simulink model "real_LAB4"  (R2025b)
settings: Solver=VariableStepAuto  StartTime=0.0  StopTime=10.0  RelTol=1e-3
undefined symbols (not defined in the file or in its folder): C, DiscIntNeverNeededParam, drv, gbox, K, K_e, Nu, Nx, sens, Tc, Ts, wheel
settings Model: Creator=ester  LastModifiedBy=ester

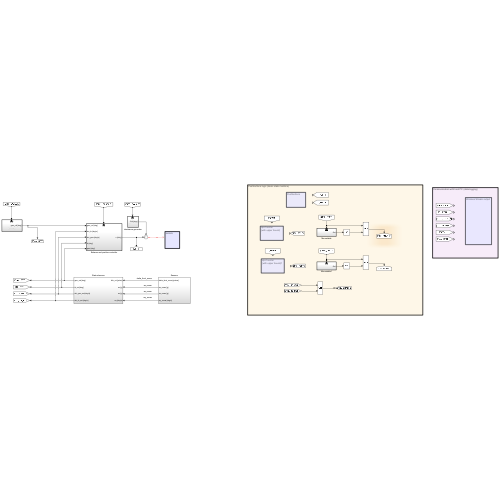
[thumbnail: Simulink's stored preview of the top-level diagram]
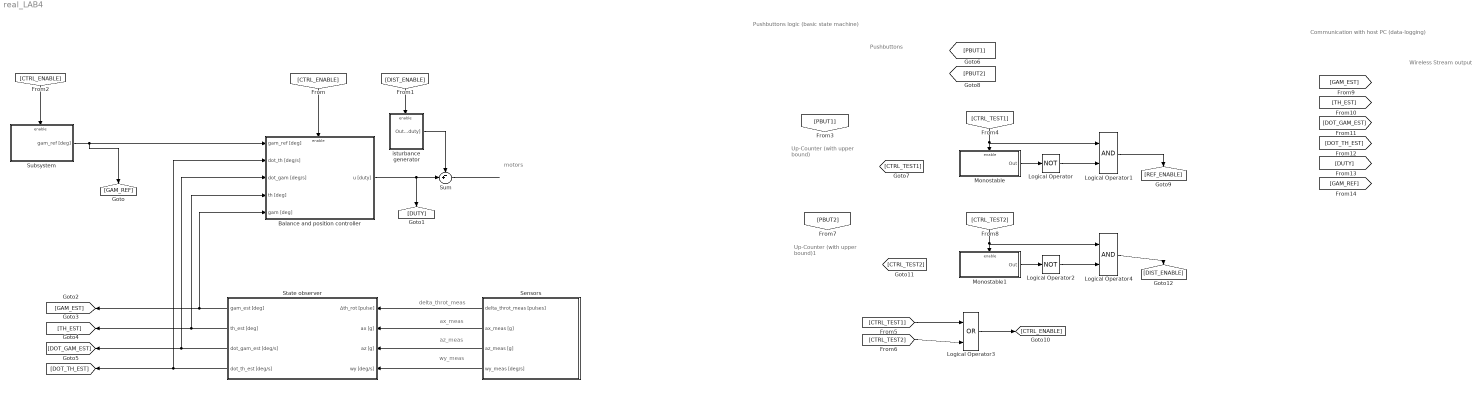
== system real_LAB4 ==
  note: Communication with host PC (data-logging)
  note: Wireless Stream output
  note: Pushbuttons logic (basic state machine)
  note: Up-Counter
      | (with upper bound)
  note: Pushbuttons
  note: motors
  note: ax_meas
  note: delta_throt_meas
  note: az_meas
  note: wy_meas
  note: Up-Counter
      | (with upper bound)1
  Balance and position controller : Subsystem
  Logical Operator : Logic  Operator=NOT  AllPortsSameDT=off  OutDataTypeStr=boolean
  Logical Operator1 : Logic  AllPortsSameDT=off  OutDataTypeStr=boolean
  Logical Operator2 : Logic  Operator=NOT  AllPortsSameDT=off  OutDataTypeStr=boolean
  Logical Operator3 : Logic  Operator=OR  AllPortsSameDT=off  OutDataTypeStr=boolean
  Logical Operator4 : Logic  AllPortsSameDT=off  OutDataTypeStr=boolean
  Monostable : Subsystem
  Monostable1 : Subsystem
  Sensors : Subsystem
  State observer : Subsystem
  Subsystem : Subsystem
  Sum : Sum  Inputs=-+|
  isturbance generator : Subsystem
  wires:
  Subsystem/1(gam_ref [deg]) -> [GAM_REF], Balance and position controller/1(gam_ref [deg])
  Balance and position controller/1(u [duty]) -> [DUTY], Sum/2
  isturbance generator/1(Out [duty]) -> Sum/1
  [DIST_ENABLE] -> isturbance generator/Enable
  [CTRL_ENABLE] -> Subsystem/Enable
  [CTRL_ENABLE] -> Balance and position controller/Enable
  Sum/1 -> ?
  Sensors/3(az_meas [g]) -> State observer/3(az [g])
  Sensors/4(wy_meas [deg/s]) -> State observer/4(wy [deg/s])
  Sensors/2(ax_meas [g]) -> State observer/2(ax [g])
  Sensors/1(delta_throt_meas [pulses]) -> State observer/1(Δth_rot [pulse])
  State observer/2(th_est [deg]) -> [TH_EST], Balance and position controller/4(th [deg])
  State observer/3(dot_gam_est [deg/s]) -> Balance and position controller/3(dot_gam [deg/s]), [DOT_GAM_EST]
  State observer/4(dot_th_est [deg/s]) -> [DOT_TH_EST], Balance and position controller/2(dot_th [deg/s])
  [CTRL_TEST1] -> Logical Operator1/1, Monostable/Enable
  Logical Operator/1 -> Logical Operator1/2
  Monostable/1(Out) -> Logical Operator/1
  Logical Operator1/1 -> [REF_ENABLE]
  Logical Operator3/1 -> [CTRL_ENABLE]
  [CTRL_TEST1] -> Logical Operator3/1
  [CTRL_TEST2] -> Logical Operator3/2
  Logical Operator4/1 -> [DIST_ENABLE]
  Logical Operator2/1 -> Logical Operator4/2
  Monostable1/1(Out) -> Logical Operator2/1
  [CTRL_TEST2] -> Logical Operator4/1, Monostable1/Enable
  State observer/1(gam_est [deg]) -> [GAM_EST], Balance and position controller/5(gam [deg])

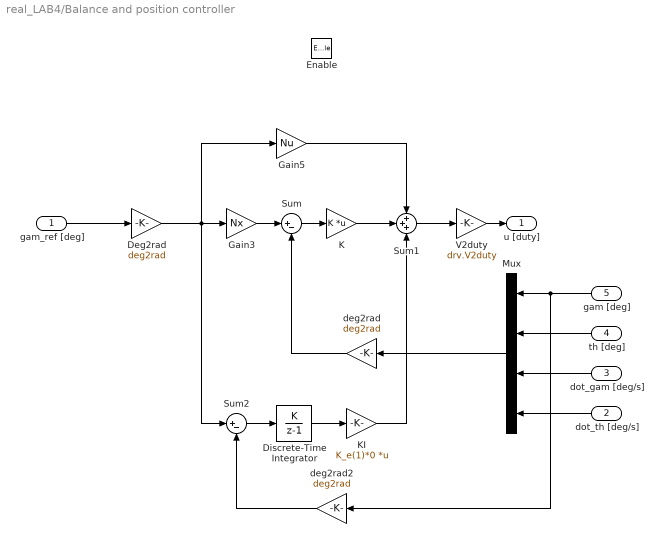
== system real_LAB4/Balance and position controller ==
  gam_ref [deg] : Inport
  dot_th [deg/s] : Inport  Port=2
  dot_gam [deg/s] : Inport  Port=3
  th [deg] : Inport  Port=4
  gam [deg] : Inport  Port=5
  Enable : EnablePort
  Deg2rad : Gain  Gain=deg2rad
  Discrete-Time Integrator : DiscreteIntegrator  IntegratorMethod=Accumulation: Forward Euler  SampleTime=Ts  ICPrevOutput=DiscIntNeverNeededParam  ICPrevScaledInput=DiscIntNeverNeededParam
  Gain3 : Gain  Gain=Nx
  Gain5 : Gain  Gain=Nu
  K : Gain  Gain=K  Multiplication=Matrix(K*u)
  KI : Gain  Gain=K_e(1)*0  Multiplication=Matrix(K*u)
  Mux : Mux
  Sum : Sum  Inputs=|+-
  Sum1 : Sum  Inputs=+++
  Sum2 : Sum  Inputs=|+-
  V2duty : Gain  Gain=drv.V2duty
  deg2rad : Gain  Gain=deg2rad
  deg2rad2 : Gain  Gain=deg2rad
  u [duty] : Outport
  wires:
  Gain5/1 -> Sum1/1
  Sum1/1 -> V2duty/1
  dot_gam [deg/s]/1 -> Mux/3
  Deg2rad/1 -> Sum2/1, Gain5/1, Gain3/1
  gam_ref [deg]/1 -> Deg2rad/1
  Gain3/1 -> Sum/1
  th [deg]/1 -> Mux/2
  V2duty/1 -> u [duty]/1
  deg2rad2/1 -> Sum2/2
  KI/1 -> Sum1/3
  deg2rad/1 -> Sum/2
  Mux/1 -> deg2rad/1
  K/1 -> Sum1/2
  Sum/1 -> K/1
  dot_th [deg/s]/1 -> Mux/4
  Sum2/1 -> Discrete-Time Integrator/1
  gam [deg]/1 -> Mux/1, deg2rad2/1
  Discrete-Time Integrator/1 -> KI/1

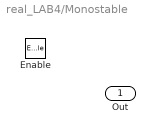
== system real_LAB4/Monostable ==
  Enable : EnablePort
  Out : Outport

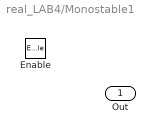
== system real_LAB4/Monostable1 ==
  Enable : EnablePort
  Out : Outport

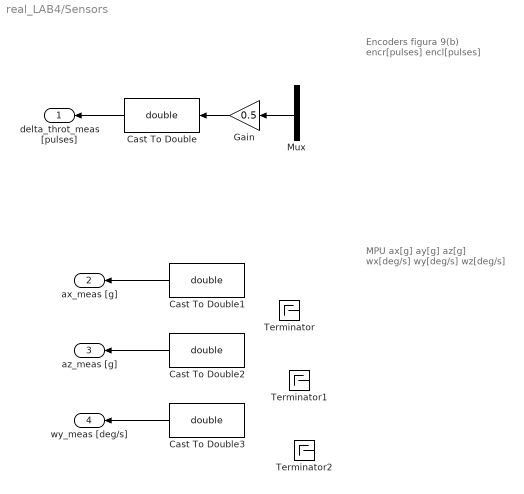
== system real_LAB4/Sensors ==
  note: Encoders figura 9(b)
      |
      | encr[pulses]
      |
      | encl[pulses]
  note: MPU
      |
      | ax[g]
      |
      | ay[g]
      |
      |
      | az[g]
      |
      | wx[deg/s]
      |
      |
      | wy[deg/s]
      |
      | wz[deg/s]
  Cast To Double{,1..3} (4 alike) : DataTypeConversion  OutDataTypeStr=double  SaturateOnIntegerOverflow=off  RndMeth=Floor
  Gain : Gain  Gain=0.5
  Mux : Mux  Inputs=2
  Terminator : Terminator
  Terminator1 : Terminator
  Terminator2 : Terminator
  delta_throt_meas [pulses] : Outport
  ax_meas [g] : Outport  Port=2
  az_meas [g] : Outport  Port=3
  wy_meas [deg/s] : Outport  Port=4
  wires:
  ? -> Terminator2/1
  ? -> Mux/1
  ? -> Cast To Double1/1
  ? -> Mux/2
  ? -> Terminator/1
  ? -> Cast To Double3/1
  ? -> Terminator1/1
  Gain/1 -> Cast To Double/1
  Mux/1 -> Gain/1
  Cast To Double/1 -> delta_throt_meas [pulses]/1
  Cast To Double1/1 -> ax_meas [g]/1
  Cast To Double3/1 -> wy_meas [deg/s]/1
  Cast To Double2/1 -> az_meas [g]/1
  ? -> Cast To Double2/1

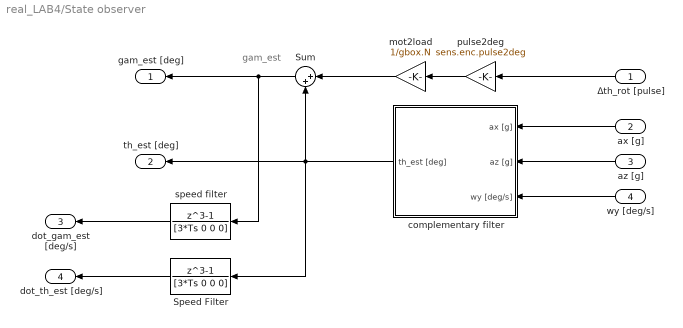
== system real_LAB4/State observer ==
  note: gam_est
  Δth_rot [pulse] : Inport
  ax [g] : Inport  Port=2
  az [g] : Inport  Port=3
  wy [deg/s] : Inport  Port=4
  Speed Filter : DiscreteTransferFcn  Numerator=[1 0 0 -1]  Denominator=[3*Ts 0 0 0]
  Sum : Sum  Inputs=|++
  complementary filter : Subsystem
  mot2load : Gain  Gain=1/gbox.N
  pulse2deg : Gain  Gain=sens.enc.pulse2deg
  speed filter : DiscreteTransferFcn  Numerator=[1 0 0 -1]  Denominator=[3*Ts 0 0 0]
  gam_est [deg] : Outport
  th_est [deg] : Outport  Port=2
  dot_gam_est [deg/s] : Outport  Port=3
  dot_th_est [deg/s] : Outport  Port=4
  wires:
  Δth_rot [pulse]/1 -> pulse2deg/1
  az [g]/1 -> complementary filter/2(az [g])
  complementary filter/1(th_est [deg]) -> Speed Filter/1, th_est [deg]/1, Sum/2
  wy [deg/s]/1 -> complementary filter/3(wy [deg/s])
  speed filter/1 -> dot_gam_est [deg/s]/1
  Sum/1 -> gam_est [deg]/1, speed filter/1
  pulse2deg/1 -> mot2load/1
  mot2load/1 -> Sum/1
  ax [g]/1 -> complementary filter/1(ax [g])
  Speed Filter/1 -> dot_th_est [deg/s]/1

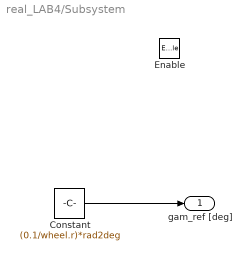
== system real_LAB4/Subsystem ==
  Enable : EnablePort
  "Constant " : Constant  Value=(0.1/wheel.r)*rad2deg  SampleTime=Ts
  gam_ref [deg] : Outport
  wires:
  "Constant "/1 -> gam_ref [deg]/1

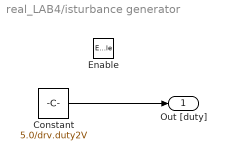
== system real_LAB4/isturbance generator ==
  Enable : EnablePort
  "Constant " : Constant  Value=5.0/drv.duty2V  SampleTime=Ts
  Out [duty] : Outport
  wires:
  "Constant "/1 -> Out [duty]/1

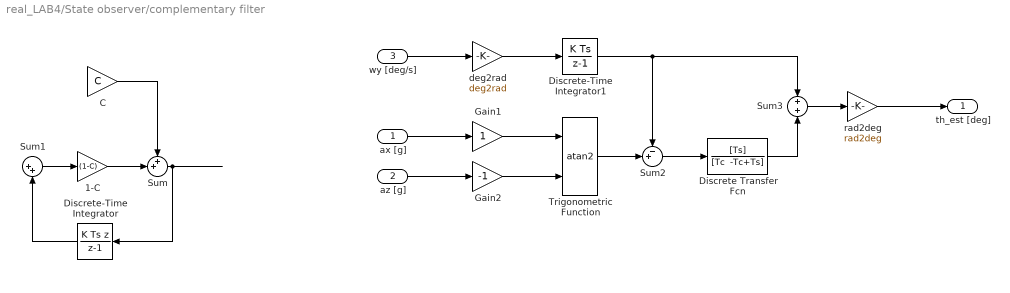
== system real_LAB4/State observer/complementary filter ==
  ax [g] : Inport
  az [g] : Inport  Port=2
  wy [deg/s] : Inport  Port=3
  1-C : Gain  Gain=(1-C)
  C : Gain  Gain=C
  Discrete Transfer Fcn : DiscreteTransferFcn  Numerator=[Ts]  Denominator="[Tc  -Tc+Ts]"
  Discrete-Time Integrator : DiscreteIntegrator  IntegratorMethod=Integration: Backward Euler  gainval=1  SampleTime=Ts  ICPrevOutput=DiscIntNeverNeededParam  ICPrevScaledInput=DiscIntNeverNeededParam
  Discrete-Time Integrator1 : DiscreteIntegrator  SampleTime=Ts  ICPrevOutput=DiscIntNeverNeededParam  ICPrevScaledInput=DiscIntNeverNeededParam
  Gain1 : Gain
  Gain2 : Gain  Gain=-1
  Sum : Sum  Inputs=++|
  Sum1 : Sum  Inputs=|++
  Sum2 : Sum  Inputs=-+|
  Sum3 : Sum  Inputs=+|+
  Trigonometric Function : Trigonometry  Operator=atan2
  deg2rad : Gain  Gain=deg2rad
  rad2deg : Gain  Gain=rad2deg
  th_est [deg] : Outport
  wires:
  Gain2/1 -> Trigonometric Function/2
  Gain1/1 -> Trigonometric Function/1
  wy [deg/s]/1 -> deg2rad/1
  az [g]/1 -> Gain2/1
  ax [g]/1 -> Gain1/1
  rad2deg/1 -> th_est [deg]/1
  Sum3/1 -> rad2deg/1
  ? -> C/1
  C/1 -> Sum/1
  1-C/1 -> Sum/2
  Discrete-Time Integrator/1 -> Sum1/2
  Sum/1 -> Discrete-Time Integrator/1
  Sum1/1 -> 1-C/1
  Trigonometric Function/1 -> Sum2/2
  Discrete Transfer Fcn/1 -> Sum3/2
  Sum2/1 -> Discrete Transfer Fcn/1
  deg2rad/1 -> Discrete-Time Integrator1/1
  Discrete-Time Integrator1/1 -> Sum2/1, Sum3/1
